simulink model "MPC_lateralStability_firstProg"  (R2019a)
settings: Solver=VariableStepAuto  StartTime=0.0  StopTime=10.0  RelTol=1e-3
values from neighbouring files (symbols this model uses):
  C = eye(4)    [model_generate.m]
undefined symbols (not defined in the file or in its folder): A, B
libraries: mpclib x1
settings Model: Creator=Shouvik Chakraborty  LastModifiedBy=Shouvik Chakraborty

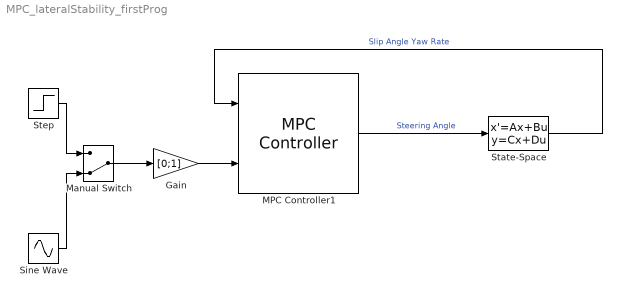
== system MPC_lateralStability_firstProg ==
  Gain : Gain  Gain=[0;1]
  MPC Controller1 : mpclib/MPC Controller  SCDEnableBlockLinearizationSpecification=on  mpcobj=mpc1  is_multiple=0  enable_value=0  return_u0=off  updateMPCinCallerWorkspace=on  md_inport=off  mv_inport=off  uref_inport=off  return_cost=off  return_mvseq=off  return_qpstatus=off  return_xseq=off  return_state=off  return_ovseq=off  state_inport=off  umin_inport=off  umax_inport=off  ymin_inport=off  ymax_inport=off  cc_inport=off  ywt_inport=off  uwt_inport=off  duwt_inport=off  rhoeps_inport=off  pm_inport=off  MaximumP=10  HorizonChoice=FixedHorizon  n_ts=0.025  n_p=10  n_mv=1  n_md=1  n_ud=0  n_mo=2  n_uo=0  BlockDataType=double  SampleTimeInherited=off  switch_inport=off
      settings: SourceProductName=MATLAB Runtime - Model Predictive Control Toolbox Addin  SourceProductBaseCode=Missing
  Manual Switch : ManualSwitch  CurrentSetting=0
  Sine Wave : Sin  SampleTime=0
  State-Space : StateSpace  A=A  B=B  C=C  D=[0;0]  InitialCondition=0
  Step : Step  SampleTime=0
  wires:
  MPC Controller1/1 -> State-Space/1  "Steering Angle"
  State-Space/1 -> MPC Controller1/1  "Slip Angle Yaw Rate"
  Manual Switch/1 -> Gain/1
  Gain/1 -> MPC Controller1/2
  Sine Wave/1 -> Manual Switch/2
  Step/1 -> Manual Switch/1
